simulink model "Scrambler_202"  (R2022a)
settings: Solver=FixedStepAuto  StartTime=0.0  StopTime=10.0  RelTol=1e-3
libraries: androidaudiovideolib x1, androiduilib x1, androidcommunicationlib x1
settings Model: Creator=mohit  LastModifiedBy=Pratyaksh Bhayre
settings OptimizationCC: EnhancedBackFolding=on  PassReuseOutputArgsThreshold=0  MaxStackSize=64  OptimizeBlockOrder=speed  DifferentSizesBufferReuse=on  OptimizationCustomize=off
settings DebuggingCC: ParameterTunabilityLossMsg=error
settings HardwareCC: ProdBitPerPointer=32  ProdBitPerSizeT=32  ProdBitPerPtrDiffT=32  ProdLargestAtomicInteger=Long  ProdLargestAtomicFloat=Double  ProdWordSize=32  ProdHWDeviceType=ARM Compatible->ARM Cortex-A (32-bit)  UseEmbeddedCoderFeatures=off  UseSimulinkCoderFeatures=off
settings ModelReferenceCC: EnableRefExpFcnMdlSchedulingChecks=off
settings SFSimCC: MATLABDynamicMemAlloc=off
settings RTWCC: SystemTargetFile=ert.tlc  HardwareBoard=Android Device  TLCOptions="-aInlineSetEventsForThisBaseRateFcn=TLC_FALSE -aSuppressMultiTaskScheduler=TLC_FALSE  -aRateBasedStepFcn=0"  TemplateMakefile=ert_default_tmf  RTWVerbose=off  Toolchain=Android SDK/NDK Tools
settings CodeAppCC: ForceParamTrailComments=on  OperatorAnnotations=on
settings ERTTargetCC: ERTCustomFileBanners=off  SupportContinuousTime=on  SupportNonInlinedSFcns=on  RemoveResetFunc=off  ModelStepFunctionPrototypeControlCompliant=off

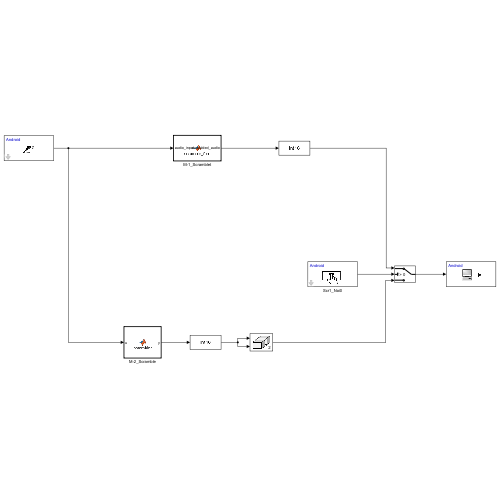
[thumbnail: Simulink's stored preview of the top-level diagram]
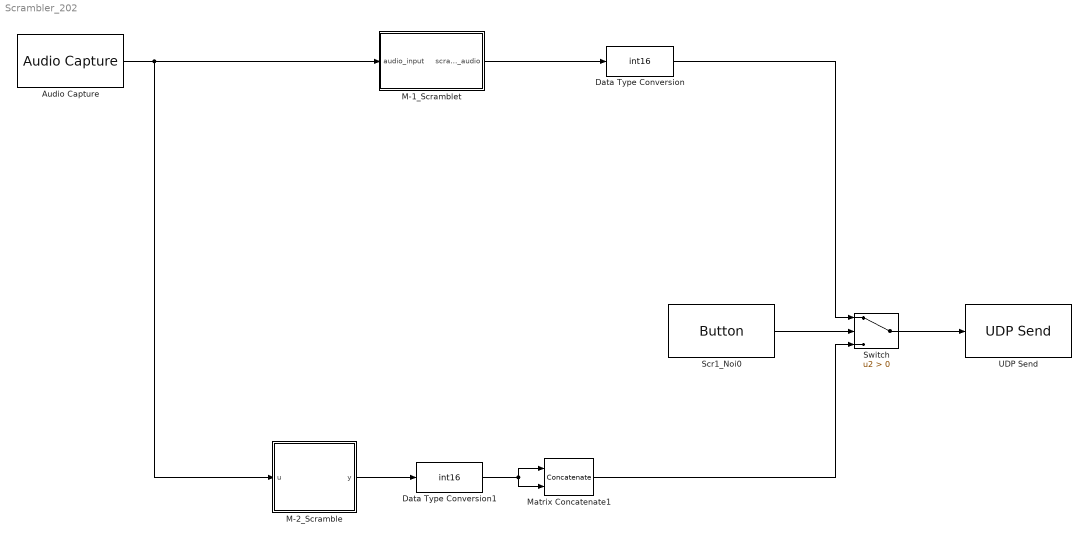
== system Scrambler_202 ==
  Audio Capture : androidaudiovideolib/Audio Capture  SampleFreq=44100  FrameSize=2205  SampleTime=0.05  SimulateUsing=Code generation  DeviceStr=0  QueueDuration=0  BlockPlatform=Android  AudioSamplingFreq=44100
      settings: SourceProductBaseCode=ANDROID
  Data Type Conversion : DataTypeConversion  OutDataTypeStr=int16  SaturateOnIntegerOverflow=off  RndMeth=Floor
  Data Type Conversion1 : DataTypeConversion  OutDataTypeStr=int16  SaturateOnIntegerOverflow=off  RndMeth=Floor
  M-1_Scramblet : MATLAB Function  TreatAsAtomicUnit=on
  M-2_Scramble : MATLAB Function  TreatAsAtomicUnit=on
  Matrix Concatenate1 : Concatenate  Mode=Multidimensional array  ConcatenateDimension=2
  Scr1_Noi0 : androiduilib/Button  ButtonState=Not pressed  ButtonId=Scrambler_202/Scr1_Noi0  State=off  SampleTime=0.1  BlockPlatform=Android
      settings: SourceProductBaseCode=ANDROID
  Switch : Switch  Criteria=u2 > Threshold  SaturateOnIntegerOverflow=off  InputSameDT=off
  UDP Send : androidcommunicationlib/UDP Send  remoteURL='10.7.26.134'  remotePort=35000  localURL='0.0.0.0'  localPortSource=Automatically determine  localPort=-1  sampletime=-1  blockPlatform=Android  separateLengthPort=0
      settings: SourceProductBaseCode=ANDROID
  wires:
  Data Type Conversion/1 -> Switch/1
  Audio Capture/1 -> M-2_Scramble/1(u), M-1_Scramblet/1(audio_input)
  M-1_Scramblet/1(scrambled_audio) -> Data Type Conversion/1
  Scr1_Noi0/1 -> Switch/2
  Switch/1 -> UDP Send/1
  M-2_Scramble/1(y) -> Data Type Conversion1/1
  Data Type Conversion1/1 -> Matrix Concatenate1/1, Matrix Concatenate1/2
  Matrix Concatenate1/1 -> Switch/3

== matlab function Scrambler_202/M-2_Scramble ==
  data: u input; y output
function y = scrambler(u)
    % Extract the first channel of the input matrix (assuming u is Nx2)
    u = u(:,1);

    % Define the bucket size
    bucketSize = 20;

    % Perform FFT on the entire signal
    fftResult = fft(u);
    avg = sum(fftResult)/length(fftResult);
    
    % Number of buckets in the entire signal
    numBuckets = floor(length(fftResult) / bucketSize);

    % Add varying noise to each element
    for i = 1:numBuckets
        % Define the range of indices for this bucket
        bucketStartIdx = (i-1) * bucketSize + 1;
        bucketEndIdx = bucketStartIdx + bucketSize - 1;

        % Add noise to each element in the bucket
        for idx = bucketStartIdx:bucketEndIdx
            noise = (idx+10) * 1e6;  % Calculate noise as index * 10,00,000
            fftResult(idx) = fftResult(idx) + noise;  % Add noise to positive frequency
            fftResult(end - idx + 2) = fftResult(end - idx + 2) + noise;  % Add noise to negative frequency
        end
    end

    % Handle any remaining elements outside of full buckets
    if mod(length(fftResult), bucketSize) ~= 0
        remainingStart = numBuckets * bucketSize + 1;
        for idx = remainingStart:length(fftResult)
            noise = (idx+10) * 1e6;  % Calculate noise as index * 10,00,000
            fftResult(idx) = fftResult(idx) + noise;  % Add noise to positive frequency
            fftResult(end - idx + 2) = fftResult(end - idx + 2) + noise;  % Add noise to negative frequency
        end
    end

    % Enforce conjugate symmetry on fftResult to ensure real output from ifft
    N = length(fftResult);
    fftResult(2:N/2) = conj(fftResult(N:-1:N/2+2));

    % Perform the inverse FFT to get the scrambled time-domain signal
    scrambledChannel = ifft(fftResult);

    % Take the real part to ensure the output is real-valued
    y = real(scrambledChannel);
end

== matlab function Scrambler_202/M-1_Scramblet ==
  data: audio_input input; scrambled_audio output
function scrambled_audio = scramble_freq(audio_input)
    % Scramble the audio input in the frequency domain with random swapping using a seed
    % audio_input: [nx2] array representing stereo audio samples
    % seed: An integer seed for generating a consistent permutation
    seed=123;
    % Pre-allocate scrambled_audio array
    scrambled_audio = zeros(size(audio_input));
    
    % Set the random seed for reproducibility
    rng(seed, 'twister');
    
    % Generate random permutation for swapping based on the seed
    n = size(audio_input, 1);
%     swap_indices = randperm(n);
    swap_indices = [n:-1:1];

    % Apply FFT to each channel separately
    freq_audio_left = fft(audio_input(:,1));
    %freq_audio_right = fft(audio_input(:,2));

    % Scramble by applying the permutation
    scrambled_freq_left = freq_audio_left(swap_indices);
    %scrambled_freq_right = freq_audio_right(swap_indices);

    % Convert scrambled frequency data back to time domain
    scrambled_audio(:,1) = real(ifft(scrambled_freq_left));
    %scrambled_audio(:,2) = real(ifft(scrambled_freq_right));
end
